simulink model "SensAdapt"  (R2013a)
settings: Solver=FixedStepDiscrete  SolverMode=SingleTasking  StartTime=0.0  StopTime=inf  FixedStep=0.01  RelTol=1e-3
libraries: SensAdapt_lib x2, simulink x1
settings Model: Creator=Beny  LastModifiedBy=User
settings DataIOCC: SaveOutput=off  SignalLogging=off  DSMLogging=off  SaveTime=off
settings OptimizationCC: ConditionallyExecuteInputs=off  InlineParams=on  InlineInvariantSignals=on  EnhancedBackFolding=on  BooleansAsBitfields=on  RollThreshold=3  StateBitsets=on  DataBitsets=on  InitFltsAndDblsToZero=on  OptimizeModelRefInitCode=on  LifeSpan=Inf
settings DebuggingCC: SignalInfNanChecking=error  SignalRangeChecking=error  ReadBeforeWriteMsg=DisableAll  WriteAfterWriteMsg=DisableAll  WriteAfterReadMsg=DisableAll  SaveWithParameterizedLinksMsg=error  UnderspecifiedInitializationDetection=Simplified  DiscreteInheritContinuousMsg=error  MultiTaskDSMMsg=warning  SingleTaskRateTransMsg=warning  TasksWithSamePriorityMsg=none  SigSpecEnsureSampleTimeMsg=error  CheckMatrixSingularityMsg=error  IntegerOverflowMsg=error  ParameterUnderflowMsg=error  ParameterPrecisionLossMsg=error  ParameterTunabilityLossMsg=error  FixptConstOverflowMsg=warning  UnderSpecifiedDataTypeMsg=error  UnnecessaryDatatypeConvMsg=warning  VectorMatrixConversionMsg=error  FcnCallInpInsideContextMsg=EnableAllAsWarning  UnconnectedInputMsg=error  UnconnectedOutputMsg=error  UnconnectedLineMsg=error  UniqueDataStoreMsg=error  BusObjectLabelMismatch=error  RootOutportRequireBusObject=error  ModelReferenceIOMsg=error  ModelReferenceIOMismatchMessage=error  ModelReferenceCSMismatchMessage=warning  ModelReferenceDataLoggingMessage=error  StrictBusMsg=ErrorOnBusTreatedAsVector  SFUnexpectedBacktrackingDiag=error  SFInvalidInputDataAccessInChartInitDiag=error  SFNoUnconditionalDefaultTransitionDiag=error  SFTransitionOutsideNaturalParentDiag=error
settings HardwareCC: ProdLargestAtomicInteger=Long  ProdLargestAtomicFloat=Double  ProdEndianess=LittleEndian  ProdHWDeviceType=ARM Compatible->ARM Cortex
settings ModelReferenceCC: ModelReferenceNumInstancesAllowed=Single  ModelReferencePassRootInputsByReference=off
settings RTWCC: SystemTargetFile=ert.tlc  GenCodeOnly=on  TemplateMakefile=ert_default_tmf  Description=Embedded Coder  GenerateReport=on  TLCAssert=on  ProcessScript=ert_make_rtw_hook  IncludeHyperlinkInReport=on  LaunchReport=on  GenerateTraceInfo=on  GenerateTraceReport=on  GenerateTraceReportSl=on  GenerateTraceReportSf=on  GenerateTraceReportEml=on
settings CodeAppCC: ForceParamTrailComments=on  IgnoreCustomStorageClasses=off  IgnoreTestpoints=on  MaxIdLength=64  SimulinkDataObjDesc=on  SFDataObjDesc=on  MangleLength=4  CustomSymbolStrType=$N$R$M  CustomSymbolStrFcnArg=rtu_$I$N$M  DefineNamingRule=UpperCase  InsertBlockDesc=on  MATLABSourceComments=on  InternalIdentifier=Classic  ReqsInCode=on
settings ERTTargetCC: CodeReplacementLibrary=C89/C90 (ANSI)  IncludeMdlTerminateFcn=off  SuppressErrorStatus=on  ParenthesesLevel=Maximum  ERTCustomFileTemplate=example_file_process.tlc  PreserveExpressionOrder=on  PreserveIfCondition=on  ConvertIfToSwitch=on

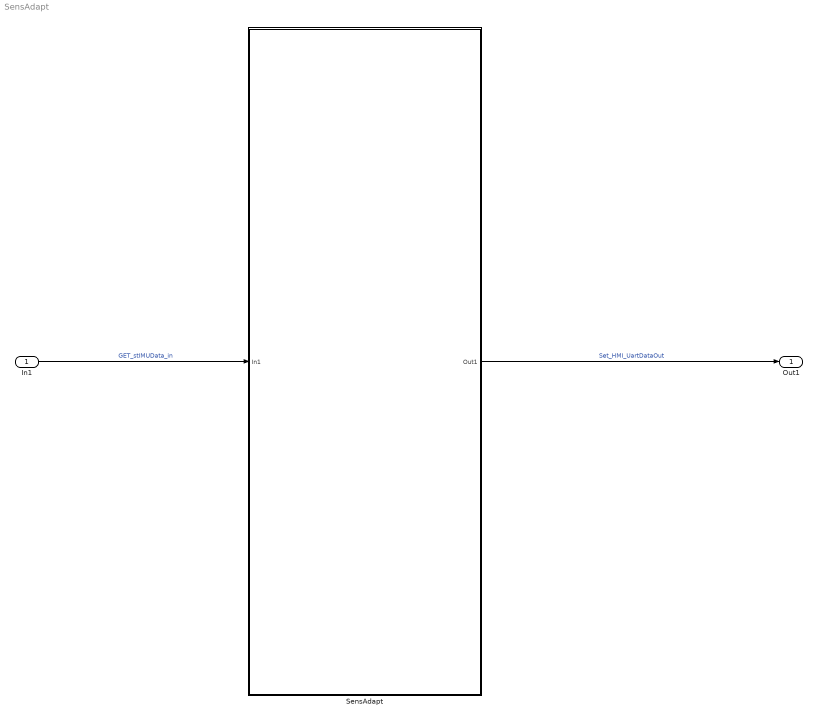
== system SensAdapt ==
  In1 : Inport  OutDataTypeStr=Bus: IMU_tstInRawData  BusOutputAsStruct=on
  SensAdapt : Subsystem
  Out1 : Outport  OutDataTypeStr=Bus: IMU_tstRawData
  wires:
  In1/1 -> SensAdapt/1(In1)  "GET_stIMUData_in"
  SensAdapt/1(Out1) -> Out1/1  "Set_HMI_UartDataOut"

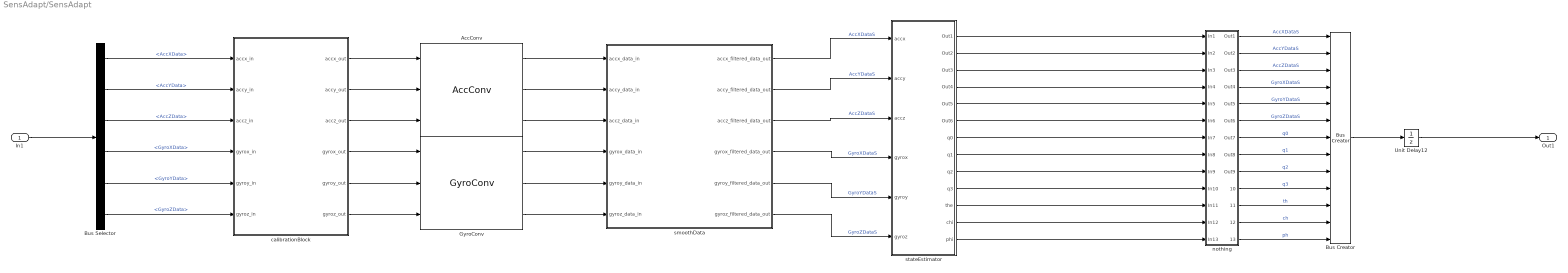
== system SensAdapt/SensAdapt ==
  In1 : Inport
  AccConv : SensAdapt_lib/AccConv  Description=acc conversion block  convParam=3
  Bus Creator : BusCreator  Inputs=13  OutDataTypeStr=Bus: IMU_tstRawData  NonVirtualBus=on
  Bus Selector : BusSelector  OutputSignals=AccXData,AccYData,AccZData,GyroXData,GyroYData,GyroZData
  GyroConv : SensAdapt_lib/GyroConv  convParam=3
  Unit Delay12 : UnitDelay  SampleTime=-1
  calibrationBlock : Subsystem  TreatAsAtomicUnit=on  mask{SENS_CalibOffsetCurve=[-710,50,467,29,-5,7]}
      mask prompts: SENS_CalibOffsetCurve "CalibOffsets"
      settings: RTWSystemCode=Nonreusable function  RTWFcnNameOpts=Use subsystem name
  nothing : Subsystem
  smoothData : Subsystem  TreatAsAtomicUnit=on
      settings: RTWSystemCode=Nonreusable function  RTWFcnNameOpts=Use subsystem name
  stateEstimator : Subsystem  mask{estimator=1}
      mask prompts: estimator "Choose state estimator"
      mask help:
      | 1 - GeneralDigits estimator
      | 2 - Madgwick estimator
      | 3 - Kalman estimator
  Out1 : Outport
  wires:
  Bus Creator/1 -> Unit Delay12/1
  Unit Delay12/1 -> Out1/1
  In1/1 -> Bus Selector/1
  AccConv/1 -> smoothData/1(accx_data_in)
  AccConv/2 -> smoothData/2(accy_data_in)
  AccConv/3 -> smoothData/3(accz_data_in)
  GyroConv/1 -> smoothData/4(gyrox_data_in)
  GyroConv/2 -> smoothData/5(gyroy_data_in)
  GyroConv/3 -> smoothData/6(gyroz_data_in)
  Bus Selector/1 -> calibrationBlock/1(accx_in)  "<AccXData>"
  Bus Selector/2 -> calibrationBlock/2(accy_in)  "<AccYData>"
  Bus Selector/3 -> calibrationBlock/3(accz_in)  "<AccZData>"
  Bus Selector/4 -> calibrationBlock/4(gyrox_in)  "<GyroXData>"
  Bus Selector/5 -> calibrationBlock/5(gyroy_in)  "<GyroYData>"
  Bus Selector/6 -> calibrationBlock/6(gyroz_in)  "<GyroZData>"
  calibrationBlock/1(accx_out) -> AccConv/1
  calibrationBlock/2(accy_out) -> AccConv/2
  calibrationBlock/3(accz_out) -> AccConv/3
  calibrationBlock/4(gyrox_out) -> GyroConv/1
  calibrationBlock/5(gyroy_out) -> GyroConv/2
  calibrationBlock/6(gyroz_out) -> GyroConv/3
  nothing/1(Out1) -> Bus Creator/1  "AccXDataS"
  nothing/3(Out3) -> Bus Creator/3  "AccZDataS"
  nothing/4(Out4) -> Bus Creator/4  "GyroXDataS"
  nothing/5(Out5) -> Bus Creator/5  "GyroYDataS"
  nothing/2(Out2) -> Bus Creator/2  "AccYDataS"
  nothing/6(Out6) -> Bus Creator/6  "GyroZDataS"
  smoothData/2(accy_filtered_data_out) -> stateEstimator/2(accy)  "AccYDataS"
  smoothData/5(gyroy_filtered_data_out) -> stateEstimator/5(gyroy)  "GyroYDataS"
  smoothData/3(accz_filtered_data_out) -> stateEstimator/3(accz)  "AccZDataS"
  smoothData/1(accx_filtered_data_out) -> stateEstimator/1(accx)  "AccXDataS"
  smoothData/4(gyrox_filtered_data_out) -> stateEstimator/4(gyrox)  "GyroXDataS"
  smoothData/6(gyroz_filtered_data_out) -> stateEstimator/6(gyroz)  "GyroZDataS"
  nothing/10(Out10) -> Bus Creator/10  "q3"
  nothing/9(Out9) -> Bus Creator/9  "q2"
  nothing/8(Out8) -> Bus Creator/8  "q1"
  nothing/7(Out7) -> Bus Creator/7  "q0"
  nothing/11(Out11) -> Bus Creator/11  "th"
  nothing/12(Out12) -> Bus Creator/12  "ch"
  nothing/13(Out13) -> Bus Creator/13  "ph"
  stateEstimator/6(Out6) -> nothing/6(In6)
  stateEstimator/5(Out5) -> nothing/5(In5)
  stateEstimator/7(q0) -> nothing/7(In7)
  stateEstimator/4(Out4) -> nothing/4(In4)
  stateEstimator/8(q1) -> nothing/8(In8)
  stateEstimator/9(q2) -> nothing/9(In9)
  stateEstimator/3(Out3) -> nothing/3(In3)
  stateEstimator/10(q3) -> nothing/10(In10)
  stateEstimator/2(Out2) -> nothing/2(In2)
  stateEstimator/1(Out1) -> nothing/1(In1)
  stateEstimator/11(the) -> nothing/11(In11)
  stateEstimator/12(chi) -> nothing/12(In12)
  stateEstimator/13(phi) -> nothing/13(In13)

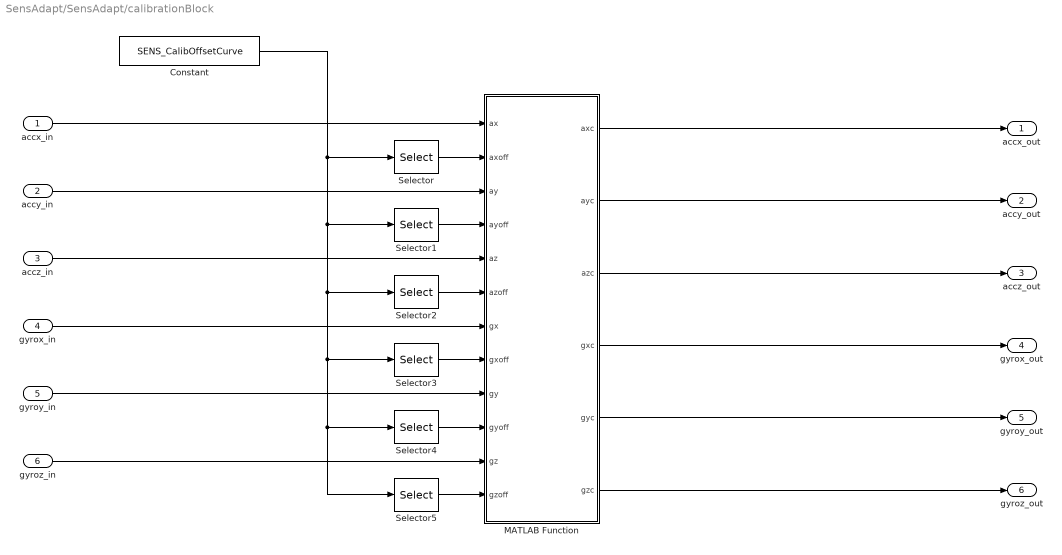
== system SensAdapt/SensAdapt/calibrationBlock ==
  accx_in : Inport
  accy_in : Inport  Port=2
  accz_in : Inport  Port=3
  gyrox_in : Inport  Port=4
  gyroy_in : Inport  Port=5
  gyroz_in : Inport  Port=6
  Constant : Constant  Value=SENS_CalibOffsetCurve  OutDataTypeStr=double
  MATLAB Function : MATLAB Function  TreatAsAtomicUnit=on
  Selector : Selector  IndexMode=Zero-based  InputPortWidth=6  IndexOptions=Index vector (dialog)  Indices=0  OutputSizes=1
  Selector1 : Selector  IndexMode=Zero-based  InputPortWidth=6  IndexOptions=Index vector (dialog)  Indices=1  OutputSizes=1
  Selector2 : Selector  IndexMode=Zero-based  InputPortWidth=6  IndexOptions=Index vector (dialog)  Indices=2  OutputSizes=1
  Selector3 : Selector  IndexMode=Zero-based  InputPortWidth=6  IndexOptions=Index vector (dialog)  Indices=3  OutputSizes=1
  Selector4 : Selector  IndexMode=Zero-based  InputPortWidth=6  IndexOptions=Index vector (dialog)  Indices=4  OutputSizes=1
  Selector5 : Selector  IndexMode=Zero-based  InputPortWidth=6  IndexOptions=Index vector (dialog)  Indices=5  OutputSizes=1
  accx_out : Outport  OutDataTypeStr=double  InitialOutput=0
  accy_out : Outport  Port=2  OutDataTypeStr=double  InitialOutput=0  LockScale=on
  accz_out : Outport  Port=3  OutDataTypeStr=double  InitialOutput=0
  gyrox_out : Outport  Port=4  OutDataTypeStr=double  InitialOutput=0
  gyroy_out : Outport  Port=5  OutDataTypeStr=double  InitialOutput=0
  gyroz_out : Outport  Port=6  OutDataTypeStr=double  InitialOutput=0
  wires:
  MATLAB Function/1(axc) -> accx_out/1
  MATLAB Function/2(ayc) -> accy_out/1
  MATLAB Function/3(azc) -> accz_out/1
  MATLAB Function/4(gxc) -> gyrox_out/1
  MATLAB Function/5(gyc) -> gyroy_out/1
  MATLAB Function/6(gzc) -> gyroz_out/1
  accy_in/1 -> MATLAB Function/3(ay)
  gyrox_in/1 -> MATLAB Function/7(gx)
  gyroz_in/1 -> MATLAB Function/11(gz)
  accz_in/1 -> MATLAB Function/5(az)
  gyroy_in/1 -> MATLAB Function/9(gy)
  accx_in/1 -> MATLAB Function/1(ax)
  Constant/1 -> Selector5/1, Selector4/1, Selector3/1, Selector2/1, Selector1/1, Selector/1
  Selector/1 -> MATLAB Function/2(axoff)
  Selector1/1 -> MATLAB Function/4(ayoff)
  Selector2/1 -> MATLAB Function/6(azoff)
  Selector3/1 -> MATLAB Function/8(gxoff)
  Selector4/1 -> MATLAB Function/10(gyoff)
  Selector5/1 -> MATLAB Function/12(gzoff)

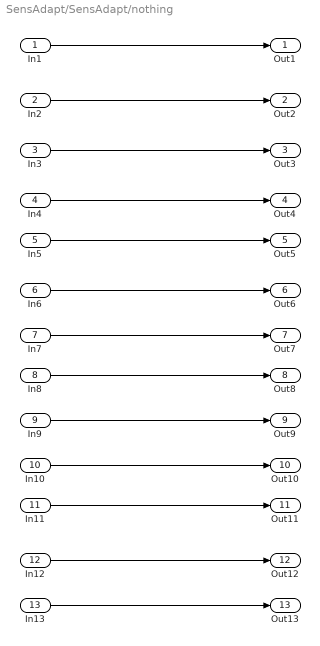
== system SensAdapt/SensAdapt/nothing ==
  In1 : Inport
  In2 : Inport  Port=2
  In3 : Inport  Port=3
  In4 : Inport  Port=4
  In5 : Inport  Port=5
  In6 : Inport  Port=6
  In7 : Inport  Port=7
  In8 : Inport  Port=8
  In9 : Inport  Port=9
  In10 : Inport  Port=10
  In11 : Inport  Port=11
  In12 : Inport  Port=12
  In13 : Inport  Port=13
  Out1 : Outport
  Out2 : Outport  Port=2
  Out3 : Outport  Port=3
  Out4 : Outport  Port=4
  Out5 : Outport  Port=5
  Out6 : Outport  Port=6
  Out7 : Outport  Port=7
  Out8 : Outport  Port=8
  Out9 : Outport  Port=9
  Out10 : Outport  Port=10
  Out11 : Outport  Port=11
  Out12 : Outport  Port=12
  Out13 : Outport  Port=13
  wires:
  In1/1 -> Out1/1
  In2/1 -> Out2/1
  In3/1 -> Out3/1
  In4/1 -> Out4/1
  In5/1 -> Out5/1
  In6/1 -> Out6/1
  In7/1 -> Out7/1
  In8/1 -> Out8/1
  In9/1 -> Out9/1
  In10/1 -> Out10/1
  In11/1 -> Out11/1
  In12/1 -> Out12/1
  In13/1 -> Out13/1

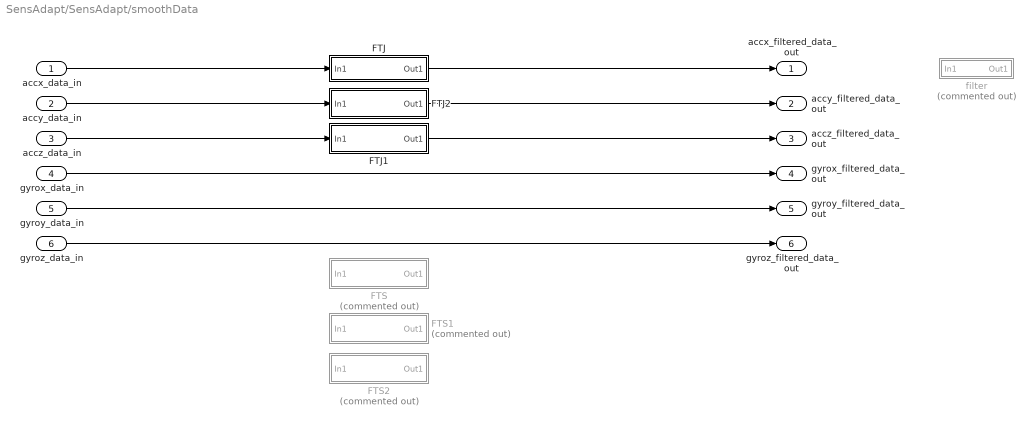
== system SensAdapt/SensAdapt/smoothData ==
  accx_data_in : Inport
  accy_data_in : Inport  Port=2
  accz_data_in : Inport  Port=3
  gyrox_data_in : Inport  Port=4
  gyroy_data_in : Inport  Port=5
  gyroz_data_in : Inport  Port=6
  FTJ : Subsystem
  FTJ1 : Subsystem
  FTJ2 : Subsystem
  FTS : Subsystem  Commented=on
  FTS1 : Subsystem  Commented=on
  FTS2 : Subsystem  Commented=on
  filter : Subsystem  Commented=on
  accx_filtered_data_out : Outport  OutDataTypeStr=double
  accy_filtered_data_out : Outport  Port=2  OutDataTypeStr=double
  accz_filtered_data_out : Outport  Port=3  OutDataTypeStr=double
  gyrox_filtered_data_out : Outport  Port=4  OutDataTypeStr=double
  gyroy_filtered_data_out : Outport  Port=5  OutDataTypeStr=double
  gyroz_filtered_data_out : Outport  Port=6  OutDataTypeStr=double
  wires:
  gyroz_data_in/1 -> gyroz_filtered_data_out/1
  gyroy_data_in/1 -> gyroy_filtered_data_out/1
  gyrox_data_in/1 -> gyrox_filtered_data_out/1
  accz_data_in/1 -> FTJ1/1(In1)
  accy_data_in/1 -> FTJ2/1(In1)
  accx_data_in/1 -> FTJ/1(In1)
  FTJ/1(Out1) -> accx_filtered_data_out/1
  FTJ2/1(Out1) -> accy_filtered_data_out/1
  FTJ1/1(Out1) -> accz_filtered_data_out/1

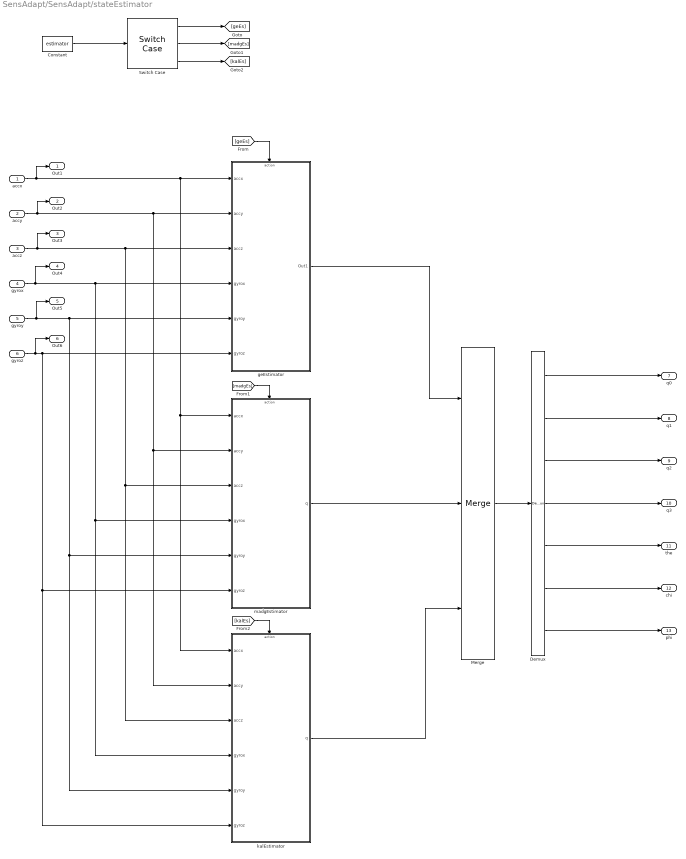
== system SensAdapt/SensAdapt/stateEstimator ==
  accx : Inport
  accy : Inport  Port=2
  accz : Inport  Port=3
  gyrox : Inport  Port=4
  gyroy : Inport  Port=5
  gyroz : Inport  Port=6
  Constant : Constant  Value=estimator
  Demux : Demux  Outputs=7
  Merge : Merge  Inputs=3  InitialOutput=0
  Switch Case : SwitchCase  CaseConditions={1,2,3}  ShowDefaultCase=off
  geEstimator : Subsystem  TreatAsAtomicUnit=on
  kalEstimator : Subsystem  TreatAsAtomicUnit=on
  madgEstimator : Subsystem  TreatAsAtomicUnit=on
  Out1 : Outport
  Out2 : Outport  Port=2
  Out3 : Outport  Port=3
  Out4 : Outport  Port=4
  Out5 : Outport  Port=5
  Out6 : Outport  Port=6
  q0 : Outport  Port=7
  q1 : Outport  Port=8
  q2 : Outport  Port=9
  q3 : Outport  Port=10
  the : Outport  Port=11
  chi : Outport  Port=12
  phi : Outport  Port=13
  wires:
  Constant/1 -> Switch Case/1
  Switch Case/1 -> [geEs]
  Switch Case/2 -> [madgEs]
  Switch Case/3 -> [kalEs]
  [madgEs] -> madgEstimator/Action
  [geEs] -> geEstimator/Action
  [kalEs] -> kalEstimator/Action
  Merge/1 -> Demux/1
  geEstimator/1(Out1) -> Merge/1
  accx/1 -> kalEstimator/1(accx), madgEstimator/1(accx), geEstimator/1(accx), Out1/1
  accy/1 -> kalEstimator/2(accy), madgEstimator/2(accy), geEstimator/2(accy), Out2/1
  accz/1 -> kalEstimator/3(accz), madgEstimator/3(accz), geEstimator/3(accz), Out3/1
  gyrox/1 -> kalEstimator/4(gyrox), madgEstimator/4(gyrox), geEstimator/4(gyrox), Out4/1
  gyroy/1 -> kalEstimator/5(gyroy), madgEstimator/5(gyroy), geEstimator/5(gyroy), Out5/1
  gyroz/1 -> Out6/1, kalEstimator/6(gyroz), madgEstimator/6(gyroz), geEstimator/6(gyroz)
  madgEstimator/1(q) -> Merge/2
  kalEstimator/1(q) -> Merge/3
  Demux/1 -> q0/1
  Demux/2 -> q1/1
  Demux/3 -> q2/1
  Demux/4 -> q3/1
  Demux/5 -> the/1
  Demux/6 -> chi/1
  Demux/7 -> phi/1

== system SensAdapt/SensAdapt/smoothData/FTJ ==
  In1 : Inport
  Add : Sum
  Constant : Constant  Value=0.2
  Constant1 : Constant  Value=0.8
  Product : Product
  Product1 : Product
  Unit Delay : UnitDelay  SampleTime=-1
  Out1 : Outport
  wires:
  Product1/1 -> Add/2
  Unit Delay/1 -> Product1/1
  Constant1/1 -> Product1/2
  Product/1 -> Add/1
  Constant/1 -> Product/2
  In1/1 -> Product/1
  Add/1 -> Unit Delay/1, Out1/1

== system SensAdapt/SensAdapt/smoothData/FTJ1 ==
  In1 : Inport
  Add : Sum
  Constant : Constant  Value=0.2
  Constant1 : Constant  Value=0.8
  Product : Product
  Product1 : Product
  Unit Delay : UnitDelay  SampleTime=-1
  Out1 : Outport
  wires:
  Add/1 -> Out1/1, Unit Delay/1
  In1/1 -> Product/1
  Constant/1 -> Product/2
  Product/1 -> Add/1
  Constant1/1 -> Product1/2
  Unit Delay/1 -> Product1/1
  Product1/1 -> Add/2

== system SensAdapt/SensAdapt/smoothData/FTJ2 ==
  In1 : Inport
  Add : Sum
  Constant : Constant  Value=0.2
  Constant1 : Constant  Value=0.8
  Product : Product
  Product1 : Product
  Unit Delay : UnitDelay  SampleTime=-1
  Out1 : Outport
  wires:
  Product1/1 -> Add/2
  Unit Delay/1 -> Product1/1
  Constant1/1 -> Product1/2
  Product/1 -> Add/1
  Constant/1 -> Product/2
  In1/1 -> Product/1
  Add/1 -> Unit Delay/1, Out1/1

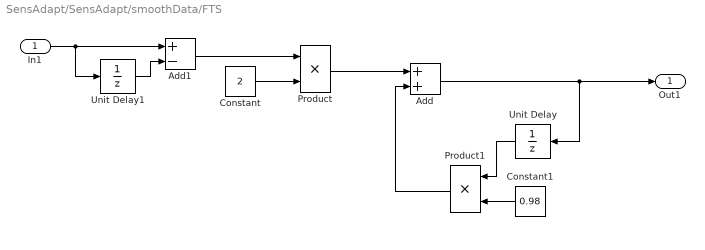
== system SensAdapt/SensAdapt/smoothData/FTS ==
  In1 : Inport
  Add : Sum
  Add1 : Sum  Inputs=+-
  Constant : Constant  Value=2
  Constant1 : Constant  Value=0.98
  Product : Product
  Product1 : Product
  Unit Delay : UnitDelay  SampleTime=-1
  Unit Delay1 : UnitDelay  SampleTime=-1
  Out1 : Outport
  wires:
  Add/1 -> Out1/1, Unit Delay/1
  Add1/1 -> Product/1
  Unit Delay1/1 -> Add1/2
  In1/1 -> Add1/1, Unit Delay1/1
  Constant/1 -> Product/2
  Product/1 -> Add/1
  Constant1/1 -> Product1/2
  Unit Delay/1 -> Product1/1
  Product1/1 -> Add/2

== system SensAdapt/SensAdapt/smoothData/FTS1 ==
  In1 : Inport
  Add : Sum
  Add1 : Sum  Inputs=+-
  Constant : Constant  Value=2
  Constant1 : Constant  Value=0.98
  Product : Product
  Product1 : Product
  Unit Delay : UnitDelay  SampleTime=-1
  Unit Delay1 : UnitDelay  SampleTime=-1
  Out1 : Outport
  wires:
  Product1/1 -> Add/2
  Unit Delay/1 -> Product1/1
  Constant1/1 -> Product1/2
  Product/1 -> Add/1
  Constant/1 -> Product/2
  In1/1 -> Unit Delay1/1, Add1/1
  Unit Delay1/1 -> Add1/2
  Add1/1 -> Product/1
  Add/1 -> Unit Delay/1, Out1/1

== system SensAdapt/SensAdapt/smoothData/FTS2 ==
  In1 : Inport
  Add : Sum
  Add1 : Sum  Inputs=+-
  Constant : Constant  Value=2
  Constant1 : Constant  Value=0.98
  Product : Product
  Product1 : Product
  Unit Delay : UnitDelay  SampleTime=-1
  Unit Delay1 : UnitDelay  SampleTime=-1
  Out1 : Outport
  wires:
  Add/1 -> Out1/1, Unit Delay/1
  Add1/1 -> Product/1
  Unit Delay1/1 -> Add1/2
  In1/1 -> Add1/1, Unit Delay1/1
  Constant/1 -> Product/2
  Product/1 -> Add/1
  Constant1/1 -> Product1/2
  Unit Delay/1 -> Product1/1
  Product1/1 -> Add/2

== system SensAdapt/SensAdapt/smoothData/filter ==
  In1 : Inport
  Product : Product  Inputs=*/  OutDataTypeStr=double
  Sum of Elements : Sum  Inputs=+  AccumDataTypeStr=double  OutDataTypeStr=double
  Tapped Delay : simulink/Discrete/Tapped Delay  vinit=0  samptime=-1  NumDelays=9  DelayOrder=Oldest  includeCurrent=off
  Vector Concatenate : Concatenate
  Width : Width  DataType=uint16
  Out1 : Outport
  wires:
  Product/1 -> Out1/1
  In1/1 -> Vector Concatenate/1, Tapped Delay/1
  Tapped Delay/1 -> Vector Concatenate/2
  Vector Concatenate/1 -> Width/1, Sum of Elements/1
  Width/1 -> Product/2
  Sum of Elements/1 -> Product/1

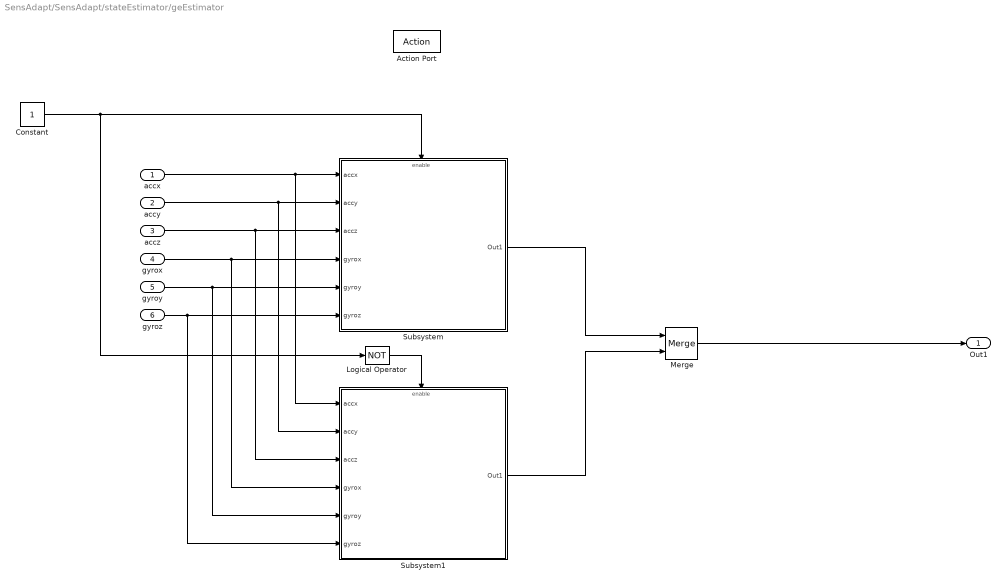
== system SensAdapt/SensAdapt/stateEstimator/geEstimator ==
  accx : Inport
  accy : Inport  Port=2
  accz : Inport  Port=3
  gyrox : Inport  Port=4
  gyroy : Inport  Port=5
  gyroz : Inport  Port=6
  Action Port : ActionPort  ActionType=case
  Constant : Constant
  Logical Operator : Logic  Operator=NOT  AllPortsSameDT=off  OutDataTypeStr=boolean
  Merge : Merge
  Subsystem : Subsystem
  Subsystem1 : Subsystem
  Out1 : Outport  InitialOutput=0
  wires:
  accx/1 -> Subsystem1/1(accx), Subsystem/1(accx)
  accy/1 -> Subsystem1/2(accy), Subsystem/2(accy)
  accz/1 -> Subsystem1/3(accz), Subsystem/3(accz)
  gyrox/1 -> Subsystem1/4(gyrox), Subsystem/4(gyrox)
  gyroy/1 -> Subsystem1/5(gyroy), Subsystem/5(gyroy)
  gyroz/1 -> Subsystem1/6(gyroz), Subsystem/6(gyroz)
  Constant/1 -> Logical Operator/1, Subsystem/Enable
  Subsystem/1(Out1) -> Merge/1
  Subsystem1/1(Out1) -> Merge/2
  Merge/1 -> Out1/1
  Logical Operator/1 -> Subsystem1/Enable

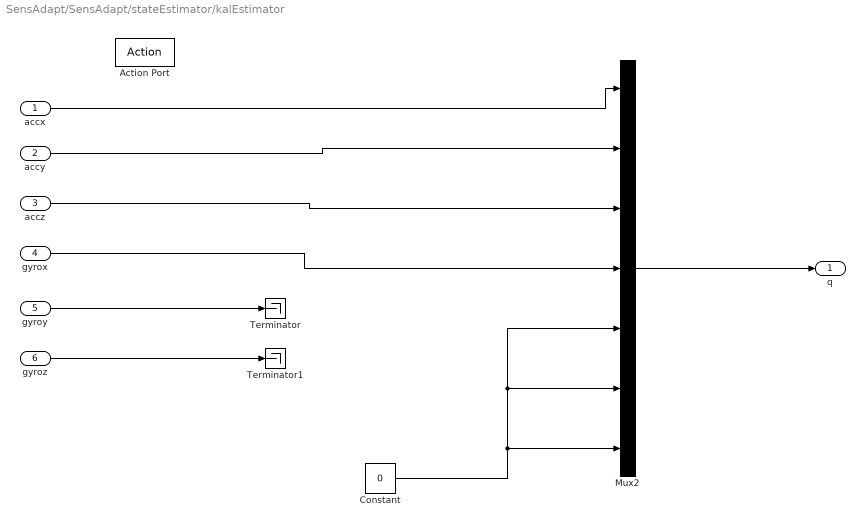
== system SensAdapt/SensAdapt/stateEstimator/kalEstimator ==
  accx : Inport
  accy : Inport  Port=2
  accz : Inport  Port=3
  gyrox : Inport  Port=4
  gyroy : Inport  Port=5
  gyroz : Inport  Port=6
  Action Port : ActionPort  ActionType=case
  Constant : Constant  Value=0
  Mux2 : Mux  Inputs=7
  Terminator : Terminator
  Terminator1 : Terminator
  q : Outport  InitialOutput=0
  wires:
  accx/1 -> Mux2/1
  accy/1 -> Mux2/2
  accz/1 -> Mux2/3
  gyrox/1 -> Mux2/4
  gyroy/1 -> Terminator/1
  gyroz/1 -> Terminator1/1
  Mux2/1 -> q/1
  Constant/1 -> Mux2/6, Mux2/5, Mux2/7

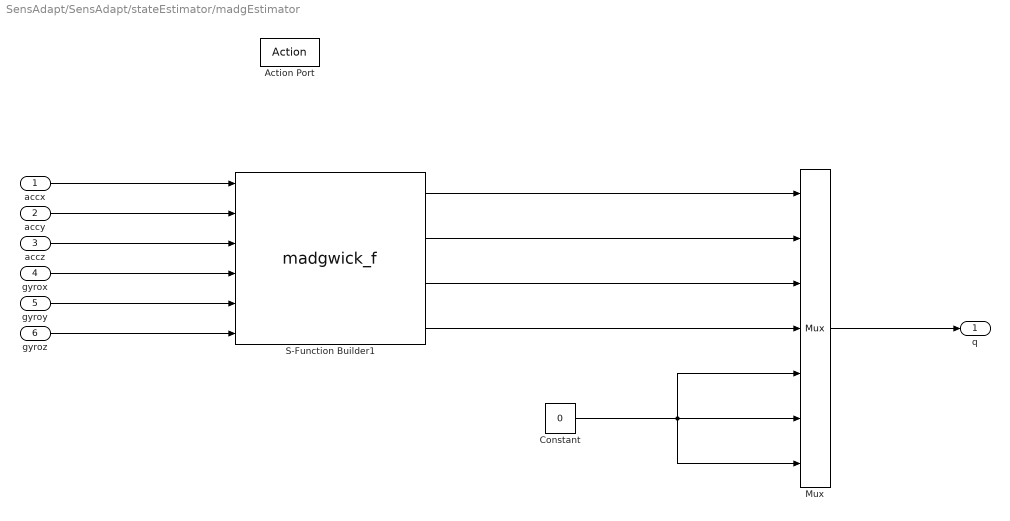
== system SensAdapt/SensAdapt/stateEstimator/madgEstimator ==
  accx : Inport
  accy : Inport  Port=2
  accz : Inport  Port=3
  gyrox : Inport  Port=4
  gyroy : Inport  Port=5
  gyroz : Inport  Port=6
  Action Port : ActionPort  ActionType=case
  Constant : Constant  Value=0
  Mux : Mux  Inputs=7
  S-Function Builder1 : S-Function  InitFcn=try, set_param(gcb,'FunctionName','madgwick_f'), end  FunctionName=madgwick_f  SFunctionModules=madgwick_f_wrapper MadgwickAHRS  EnableBusSupport=off  mask(S-Function Builder){}
      mask help: Simulink:masks:SFunctionBuilder_MD
      mask init:
      | val = [[.9  0.75 0.75 1 1 .9 .9 1]',[1 1 0.75 0.75 .9 .9 1 .9]'];try , sys = get_param(gcb,'SfunBuilderFcnName');if isempty(sys), sys = get_param(gcb,'FunctionName'); end,catch, sys = get_param(gcb,'FunctionName'); end
      settings: CopyFcn=set_param(gcbh,'LinkStatus','none')  PreSaveFcn=try, set_param(gcb,'FunctionName','madgwick_f'), end  OpenFcn=sfunctionwizard(gcbh)
      mask Display: plot(val(:,1),val(:,2)),disp(sys), port_label('input',1,'accx'), port_label('input',2,'accy'), port_label('input',3,'accz'), port_label('input',4,'gyrox'), port_label('input',5,'gyroy'), port_label('input',6,'gyroz'), port_label('output',1,'qt0'), port_label('output',2,'qt1'), port_label('output',3,'qt2'), port_label('output',4,'qt3')
  q : Outport  InitialOutput=0
  wires:
  accx/1 -> S-Function Builder1/1
  accy/1 -> S-Function Builder1/2
  accz/1 -> S-Function Builder1/3
  gyrox/1 -> S-Function Builder1/4
  gyroy/1 -> S-Function Builder1/5
  gyroz/1 -> S-Function Builder1/6
  Mux/1 -> q/1
  Constant/1 -> Mux/5, Mux/6, Mux/7
  S-Function Builder1/1 -> Mux/1
  S-Function Builder1/2 -> Mux/2
  S-Function Builder1/3 -> Mux/3
  S-Function Builder1/4 -> Mux/4

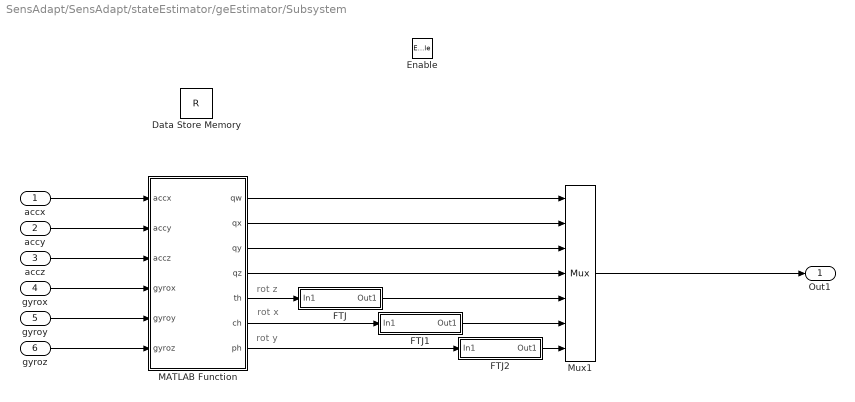
== system SensAdapt/SensAdapt/stateEstimator/geEstimator/Subsystem ==
  note: rot y
  note: rot x
  note: rot z
  accx : Inport
  accy : Inport  Port=2
  accz : Inport  Port=3
  gyrox : Inport  Port=4
  gyroy : Inport  Port=5
  gyroz : Inport  Port=6
  Enable : EnablePort
  Data Store Memory : DataStoreMemory  DataStoreName=R  ReadBeforeWriteMsg=warning  WriteAfterWriteMsg=warning  WriteAfterReadMsg=warning  InitialValue=[1 0 0;0 1 0; 0 0 1]  VectorParams1D=off  OutDataTypeStr=double
  FTJ : Subsystem
  FTJ1 : Subsystem
  FTJ2 : Subsystem
  MATLAB Function : MATLAB Function  TreatAsAtomicUnit=on
  Mux1 : Mux  Inputs=7
  Out1 : Outport
  wires:
  Mux1/1 -> Out1/1
  accx/1 -> MATLAB Function/1(accx)
  accy/1 -> MATLAB Function/2(accy)
  gyrox/1 -> MATLAB Function/4(gyrox)
  gyroy/1 -> MATLAB Function/5(gyroy)
  MATLAB Function/4(qz) -> Mux1/4
  MATLAB Function/5(th) -> FTJ/1(In1)
  MATLAB Function/3(qy) -> Mux1/3
  MATLAB Function/2(qx) -> Mux1/2
  MATLAB Function/7(ph) -> FTJ2/1(In1)
  MATLAB Function/1(qw) -> Mux1/1
  MATLAB Function/6(ch) -> FTJ1/1(In1)
  accz/1 -> MATLAB Function/3(accz)
  gyroz/1 -> MATLAB Function/6(gyroz)
  FTJ/1(Out1) -> Mux1/5
  FTJ1/1(Out1) -> Mux1/6
  FTJ2/1(Out1) -> Mux1/7

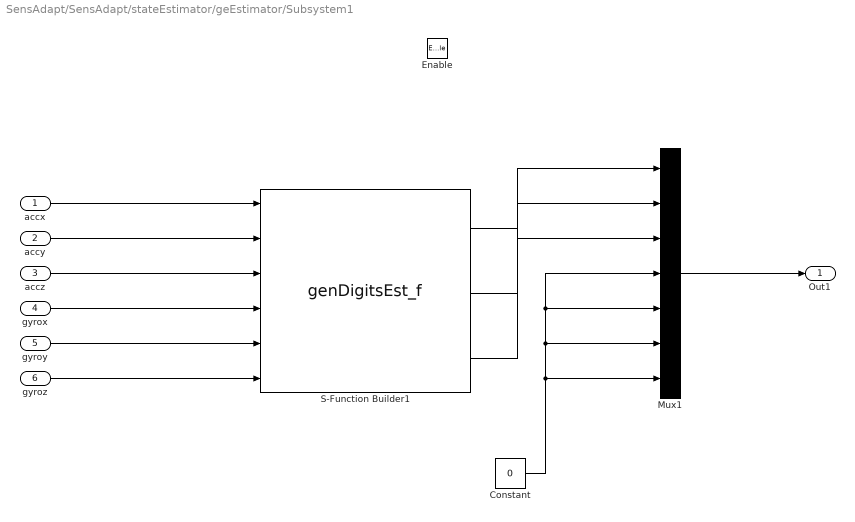
== system SensAdapt/SensAdapt/stateEstimator/geEstimator/Subsystem1 ==
  accx : Inport
  accy : Inport  Port=2
  accz : Inport  Port=3
  gyrox : Inport  Port=4
  gyroy : Inport  Port=5
  gyroz : Inport  Port=6
  Enable : EnablePort
  Constant : Constant  Value=0
  Mux1 : Mux  Inputs=7
  S-Function Builder1 : S-Function  InitFcn=try, set_param(gcb,'FunctionName','genDigitsEst_f'), end  FunctionName=genDigitsEst_f  SFunctionModules=genDigitsEst_f_wrapper genDigitsEst  EnableBusSupport=off  mask(S-Function Builder){}
      mask help: Simulink:masks:SFunctionBuilder_MD
      mask init: same as SensAdapt/SensAdapt/stateEstimator/madgEstimator/S-Function Builder1
      settings: CopyFcn=set_param(gcbh,'LinkStatus','none')  PreSaveFcn=try, set_param(gcb,'FunctionName','genDigitsEst_f'), end  OpenFcn=sfunctionwizard(gcbh)
      mask Display: plot(val(:,1),val(:,2)),disp(sys), port_label('input',1,'accx'), port_label('input',2,'accy'), port_label('input',3,'accz'), port_label('input',4,'gyrox'), port_label('input',5,'gyroy'), port_label('input',6,'gyroz'), port_label('output',1,'th'), port_label('output',2,'ch'), port_label('output',3,'ph')
  Out1 : Outport
  wires:
  Mux1/1 -> Out1/1
  accx/1 -> S-Function Builder1/1
  accy/1 -> S-Function Builder1/2
  accz/1 -> S-Function Builder1/3
  gyrox/1 -> S-Function Builder1/4
  gyroy/1 -> S-Function Builder1/5
  gyroz/1 -> S-Function Builder1/6
  S-Function Builder1/1 -> Mux1/1
  S-Function Builder1/2 -> Mux1/2
  S-Function Builder1/3 -> Mux1/3
  Constant/1 -> Mux1/7, Mux1/6, Mux1/5, Mux1/4

== system SensAdapt/SensAdapt/stateEstimator/geEstimator/Subsystem/FTJ ==
  In1 : Inport
  Add : Sum
  Constant : Constant  Value=0.2
  Constant1 : Constant  Value=0.8
  Product : Product
  Product1 : Product
  Unit Delay : UnitDelay  SampleTime=-1
  Out1 : Outport
  wires:
  Product1/1 -> Add/2
  Unit Delay/1 -> Product1/1
  Constant1/1 -> Product1/2
  Product/1 -> Add/1
  Constant/1 -> Product/2
  In1/1 -> Product/1
  Add/1 -> Unit Delay/1, Out1/1

== system SensAdapt/SensAdapt/stateEstimator/geEstimator/Subsystem/FTJ1 ==
  In1 : Inport
  Add : Sum
  Constant : Constant  Value=0.2
  Constant1 : Constant  Value=0.8
  Product : Product
  Product1 : Product
  Unit Delay : UnitDelay  SampleTime=-1
  Out1 : Outport
  wires:
  Add/1 -> Out1/1, Unit Delay/1
  In1/1 -> Product/1
  Constant/1 -> Product/2
  Product/1 -> Add/1
  Constant1/1 -> Product1/2
  Unit Delay/1 -> Product1/1
  Product1/1 -> Add/2

== system SensAdapt/SensAdapt/stateEstimator/geEstimator/Subsystem/FTJ2 ==
  In1 : Inport
  Add : Sum
  Constant : Constant  Value=0.2
  Constant1 : Constant  Value=0.8
  Product : Product
  Product1 : Product
  Unit Delay : UnitDelay  SampleTime=-1
  Out1 : Outport
  wires:
  Product1/1 -> Add/2
  Unit Delay/1 -> Product1/1
  Constant1/1 -> Product1/2
  Product/1 -> Add/1
  Constant/1 -> Product/2
  In1/1 -> Product/1
  Add/1 -> Unit Delay/1, Out1/1

== matlab function SensAdapt/stateEstimator/geEstimator/Subsystem/MATLAB Function ==
  data: qw output; qx output; qy output; qz output; accx input; th output; accy input; accz input; gyrox input; gyroy input; gyroz input; R data_store_memory; ch output; ph output
function [qw,qx,qy,qz,th,ch,ph]  = fcn(accx,accy,accz,gyrox,gyroy,gyroz)
%#codegen

global R;

%R = eye(3);
    
ts = 0.01;
k = 50;

%integration
wx = gyrox;
wy = gyroy;
wz = gyroz;

wb_vp = [0 -wz wy; wz 0 -wx;-wy wx 0];
R_test = R*(eye(3)+ ts*wb_vp);

%orthogonalization
X = R_test(:,1);
Y = R_test(:,2);

err = X' * Y;
r1 = X - err/2*Y;
r2 = Y - err/2*X;
r3 = cross(r1,r2);

Xn = 1/2*(3-r1'*r1)*r1;
Yn = 1/2*(3-r2'*r2)*r2;
Zn = 1/2*(3-r3'*r3)*r3;

R_test = [Xn,Yn,Zn];

%   sensor fusion
OZ_acc = ([accx;accy;accz]);
OZ_acc = OZ_acc/norm(OZ_acc);
OZ_gyro = R_test*[0;0;1];

wf = k*cross(OZ_gyro,OZ_acc);
W = [wx;wy;wz] - wf;

wb_vp = [0 -W(3) W(2); W(3) 0 -W(1);-W(2) W(1) 0];
R = R*(eye(3)+ ts*wb_vp);

%   orthogonalization
X = R(:,1);
Y = R(:,2);

err = X' * Y;
r1 = X - err/2*Y;
r2 = Y - err/2*X;
r3 = cross(r1,r2);

Xn = 1/2*(3-r1'*r1)*r1;
Yn = 1/2*(3-r2'*r2)*r2;
Zn = 1/2*(3-r3'*r3)*r3;

R = [Xn,Yn,Zn];

ch = asin(R(3,2));
ch2 = -asin(R(3,2))+pi;

if abs(cos(ch)) > 0.01
    ph = atan2(-R(3,1)/cos(ch),R(3,3)/cos(ch));
    th = atan2(-R(2,1)/cos(ch2),R(2,2)/cos(ch2));
    if th > pi/0.1
       th = th-2*pi; 
    end
else
    ph = 0;
    th = 0;
end

% aflare quaternioni
tr = R(1,1) + R(2,2) + R(3,3);

m00 = R(1,1);
m01 = R(1,2);
m02 = R(1,3);
m10 = R(2,1);
m11 = R(2,2);
m12 = R(2,3);
m20 = R(3,1);
m21 = R(3,2);
m22 = R(3,3);

if (tr > 0)
  S = sqrt(tr+1.0) * 2; 
  qw = 0.25 * S;
  qx = (m21 - m12) / S;
  qy = (m02 - m20) / S; 
  qz = (m10 - m01) / S; 
elseif ((m00 > m11)&&(m00 > m22))
  S = sqrt(1.0 + m00 - m11 - m22) * 2; 
  qw = (m21 - m12) / S;
  qx = 0.25 * S;
  qy = (m01 + m10) / S; 
  qz = (m02 + m20) / S; 
elseif (m11 > m22)
  S = sqrt(1.0 + m11 - m00 - m22) * 2; 
  qw = (m02 - m20) / S;
  qx = (m01 + m10) / S; 
  qy = 0.25 * S;
  qz = (m12 + m21) / S; 
 else 
  S = sqrt(1.0 + m22 - m00 - m11) * 2; 
  qw = (m10 - m01) / S;
  qx = (m02 + m20) / S;
  qy = (m12 + m21) / S;
  qz = 0.25 * S;
end

end

== matlab function SensAdapt/calibrationBlock/MATLAB Function ==
  data: axc output; ayc output; azc output; gxc output; gyc output; gzc output; ax input; axoff input; ay input; ayoff input; az input; azoff input; gx input; gxoff input; gy input; gyoff input; gz input; gzoff input
function [axc,ayc,azc,gxc,gyc,gzc] = fcn(ax,axoff,ay,ayoff,az,azoff,gx,gxoff,gy,gyoff,gz,gzoff)

axc = ax - axoff;
ayc = ay - ayoff;
azc = az - azoff;
gxc = gx - gxoff;
gyc = gy - gyoff;
gzc = gz - gzoff;


end
